simulink model "F16LQRController"  (R2023a)
settings: Solver=VariableStepAuto  StartTime=0.0  StopTime=10  RelTol=1e-3
undefined symbols (not defined in the file): A, A_lat, B, B_lat, C_lat, D_lat, Earth, f16, K, K_lat, N_bar, simplified, WGS84
libraries: aerolibfltsims x2, aerolibtransform2 x1
settings Model: Creator=GURU  LastModifiedBy=Aleyna
settings SolverCC: AlgebraicLoopSolver=TrustRegion
settings DebuggingCC: UnconnectedInputMsg=warning  UnconnectedOutputMsg=warning  UnconnectedLineMsg=warning
settings ModelReferenceCC: EnableRefExpFcnMdlSchedulingChecks=on
settings RTWCC: DLArmComputeVersion=19.05

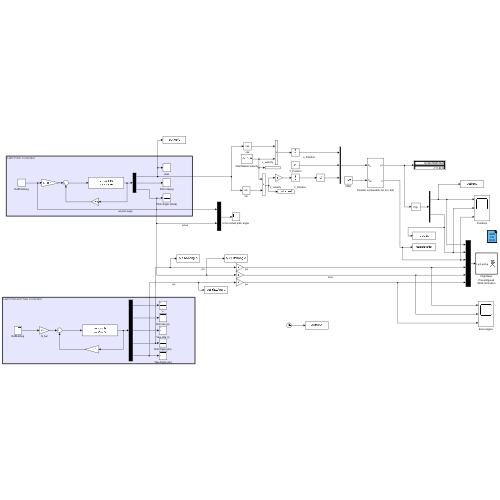
[thumbnail: Simulink's stored preview of the top-level diagram]
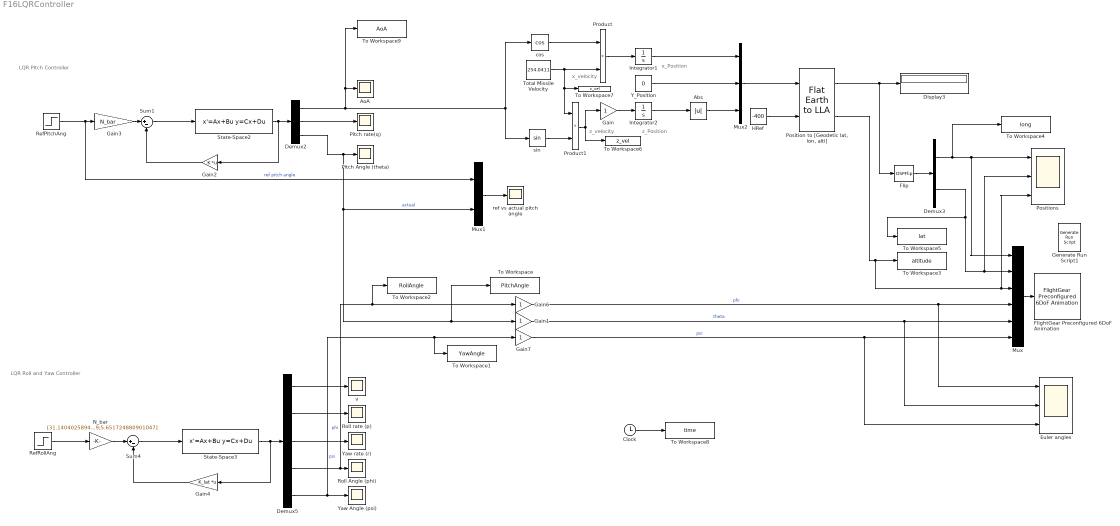
== system F16LQRController ==
  note: LQR Pitch Controller
  note: z_Position
  note: z_velocity
  note: x_velocity
  note: x_Position
  note: LQR Roll and Yaw Controller
  Abs : Abs  SaturateOnIntegerOverflow=off
  AoA : Scope
  Clock : Clock
  Demux2 : Demux  Outputs=3
  Demux3 : Demux  Outputs=2
  Demux5 : Demux  Outputs=5
  Display3 : Display
      settings: Decimation=2
  Euler angles : Scope  NumInputPorts=3
  FlightGear Preconfigured 6DoF Animation : aerolibfltsims/FlightGear Preconfigured 6DoF Animation  xFlightGearVersion=v2019.1  DestinationIpAddress=127.0.0.1  DestinationPort=5502  SampleTime=1/30  packetVersion=24
  Flip : DSPFlip
  Gain{,1,6..7} (4 alike) : Gain
  Gain2 : Gain  Gain=K  Multiplication=Matrix(K*u)
  Gain3 : Gain  Gain=N_bar
  Gain4 : Gain  Gain=K_lat  Multiplication=Matrix(K*u)
  Generate Run Script1 : aerolibfltsims/Generate Run Script  Architecture=Win64  dataFlow=Send  GeometryModelName=f16-simplified  AirportId=KSFO  RunwayId=10L  InitialAltitude=7224  InitialHeading=113  OffsetDistance=4.72  OffsetAzimuth=0  InstallScenery=off  DisableShaders=off  OriginAddress=127.0.0.1  DestinationPort=5502  OriginPort=5505  LocalAddress=127.0.0.1  OutputFileName=runfg.bat  FlightGearBaseDirectory=C:\Program Files\FlightGear 2020.3
  HRef : Constant  Value=-400
  Integrator1 : Integrator
  Integrator2 : Integrator  InitialCondition=-500
  Mux : Mux  Inputs=6
  Mux1 : Mux  Inputs=2
  Mux2 : Mux  Inputs=3
  N_bar : Gain  Gain=[31.1404025894999;5.651724880901047]
  Pitch Angle (theta) : Scope
  Pitch rate(q) : Scope
  "Position to [Geodetic lat, lon, alti]" : aerolibtransform2/Flat Earth to LLA  units=Metric (MKS)  ptype=Earth (WGS84)  F=1/298.257223563  R=6378137  refPosPort=off  LL0=[34.910 -117.8912]  psi=0
  Positions : Scope  NumInputPorts=3
  Product : Product
  Product1 : Product
  RefPitchAng : Step  Time=0  SampleTime=0
  RefRollAng : Step  Time=0  SampleTime=0
  Roll Angle (phi) : Scope
  Roll rate (p) : Scope
  State-Space2 : StateSpace  A=A  B=B  C=eye(3)  D=[0;0;0]  InitialCondition=0  ContinuousStateAttributes={'aoa', 'pitch_rate', 'pitch_angle'}
  State-Space3 : StateSpace  A=A_lat  B=B_lat  C=C_lat  D=D_lat  InitialCondition=0  ContinuousStateAttributes={'v', 'p', 'r','phi','psi'}
  Sum1 : Sum  Inputs=|+-
  Sum4 : Sum  Inputs=|+-
  To Workspace : ToWorkspace  VariableName=PitchAngle  SampleTime=-1
  To Workspace1 : ToWorkspace  VariableName=YawAngle  SampleTime=-1
  To Workspace2 : ToWorkspace  VariableName=RollAngle  SampleTime=-1
  To Workspace3 : ToWorkspace  VariableName=altitude  SampleTime=-1
  To Workspace4 : ToWorkspace  VariableName=long  SampleTime=-1
  To Workspace5 : ToWorkspace  VariableName=lat  SampleTime=-1
  To Workspace6 : ToWorkspace  VariableName=z_vel  SampleTime=-1
  To Workspace7 : ToWorkspace  VariableName=x_vel  SampleTime=-1
  To Workspace8 : ToWorkspace  VariableName=time  SampleTime=-1
  To Workspace9 : ToWorkspace  VariableName=AoA  SampleTime=-1
  Total Missile Velocity : Constant  Value=254.0411
  Y_Position : Constant  Value=0
  Yaw Angle (psi) : Scope
  Yaw rate (r) : Scope
  cos : Trigonometry  Operator=cos
  "ref vs actual pitch angle " : Scope
  sin : Trigonometry
  v : Scope
  wires:
  RefPitchAng/1 -> Mux1/1, Gain3/1  "ref pitch angle"
  Sum1/1 -> State-Space2/1
  State-Space2/1 -> Gain2/1, Demux2/1
  Demux2/3 -> Mux1/2, To Workspace/1, Gain1/1, Pitch Angle (theta)/1  "actual"
  Demux2/2 -> Pitch rate(q)/1
  "Position to [Geodetic lat, lon, alti]"/1 -> Flip/1, Display3/1
  Demux2/1 -> To Workspace9/1, AoA/1, cos/1, sin/1
  cos/1 -> Product/1
  Gain/1 -> Integrator2/1
  Mux2/1 -> "Position to [Geodetic lat, lon, alti]"/1
  Mux/1 -> FlightGear Preconfigured 6DoF Animation/1
  Integrator1/1 -> Mux2/1
  Y_Position/1 -> Mux2/2
  sin/1 -> Product1/2
  HRef/1 -> "Position to [Geodetic lat, lon, alti]"/2
  Total Missile Velocity/1 -> Product1/1, To Workspace7/1, Product/2
  Product/1 -> Integrator1/1
  Product1/1 -> Gain/1, To Workspace6/1
  Mux1/1 -> "ref vs actual pitch angle "/1
  Gain1/1 -> Euler angles/2, Mux/5  "theta"
  Gain2/1 -> Sum1/2
  Gain3/1 -> Sum1/1
  Flip/1 -> Demux3/1
  Demux5/5 -> Yaw Angle (psi)/1, Gain7/1, To Workspace1/1  "psi"
  Demux5/4 -> To Workspace2/1, Gain6/1, Roll Angle (phi)/1  "phi"
  Gain4/1 -> Sum4/2
  Demux5/2 -> Roll rate (p)/1
  State-Space3/1 -> Gain4/1, Demux5/1
  Demux5/1 -> v/1
  Demux5/3 -> Yaw rate (r)/1
  Sum4/1 -> State-Space3/1
  Gain6/1 -> Euler angles/1, Mux/4  "phi"
  Gain7/1 -> Euler angles/3, Mux/6  "psi"
  Integrator2/1 -> Abs/1
  Abs/1 -> Mux2/3
  RefRollAng/1 -> N_bar/1
  N_bar/1 -> Sum4/1
  Demux3/2 -> Positions/2, Mux/2, To Workspace5/1
  Demux3/1 -> To Workspace4/1, Positions/1, Mux/1
  "Position to [Geodetic lat, lon, alti]"/2 -> Positions/3, Mux/3, To Workspace3/1
  Clock/1 -> To Workspace8/1
